simulink model "cdif"  (R2018a)
settings: Solver=VariableStepAuto  StartTime=0.0  StopTime=1.0  RelTol=1e-3
undefined symbols (not defined in the file): A, B, C
libraries: fuzblock x1
settings Model: Creator=daniel  LastModifiedBy=daniel
settings SolverCC: ZeroCrossControl=DisableAll

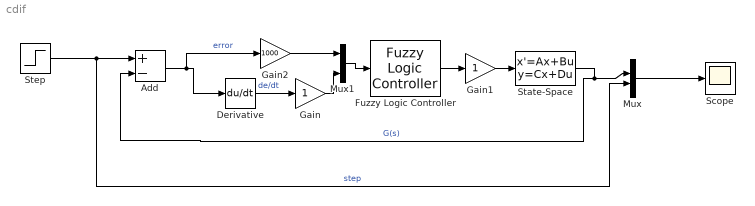
== system cdif ==
  Add : Sum  Inputs=+-
  Derivative : Derivative
  Fuzzy Logic Controller : fuzblock/Fuzzy Logic  Controller  FIS=sys  OutputSampleNumber=101  DataType=double  FuzzifiedInputs=off  RuleFiringStrengths=off  RuleOutputs=off  AggregatedOutputs=off  SimulateUsing=Interpreted execution  OutOfRangeInputValueMessage=warning  NoRuleFiredMessage=warning  EmptyOutputFuzzySetMessage=warning
  Gain : Gain
  Gain1 : Gain
  Gain2 : Gain  Gain=1000
  Mux : Mux
  Mux1 : Mux  Inputs=2
  Scope : Scope
  State-Space : StateSpace  A=A  B=B  C=C  D=0  InitialCondition=0
  Step : Step  Time=0  SampleTime=0
  wires:
  Mux/1 -> Scope/1
  Fuzzy Logic Controller/1 -> Gain1/1
  State-Space/1 -> Add/2, Mux/2  "G(s)"
  Step/1 -> Add/1, Mux/3  "step"
  Mux1/1 -> Fuzzy Logic Controller/1
  Add/1 -> Gain2/1, Derivative/1  "error"
  Gain1/1 -> State-Space/1
  Derivative/1 -> Gain/1  "de/dt"
  Gain/1 -> Mux1/2
  Gain2/1 -> Mux1/1
